simulink model "two_dof_system"  (R2019a)
settings: Solver=VariableStepAuto  StartTime=0.0  StopTime=time_span(end)  RelTol=1e-3
values from neighbouring files (symbols this model uses):
  c_f = damping    [cost_function.m]    (also in fourier_transform_two_dof_free.m = 100; two_dof_system_free_oscillations.m = 100)
  c_r = damping    [cost_function.m]    (also in fourier_transform_two_dof_free.m = 100; two_dof_system_free_oscillations.m = 100)
  j = 1000    [cost_function.m]    (also in fourier_transform_two_dof_free.m; two_dof_system_free_oscillations.m)
  k_f = 60000    [cost_function.m]    (also in fourier_transform_two_dof_free.m; two_dof_system_free_oscillations.m)
  k_r = 60000    [cost_function.m]    (also in fourier_transform_two_dof_free.m; two_dof_system_free_oscillations.m)
  l_f = 2.5    [cost_function.m]    (also in fourier_transform_two_dof_free.m; two_dof_system_free_oscillations.m = 4.5)
  l_r = 2.5    [cost_function.m]    (also in fourier_transform_two_dof_free.m; two_dof_system_free_oscillations.m)
  m = 1000    [cost_function.m]    (also in fourier_transform_two_dof_free.m; two_dof_system_free_oscillations.m)
  p_0 = 1.0    (= 1)    [cost_function.m]    (also in fourier_transform_two_dof_free.m; two_dof_system_free_oscillations.m)
  p_dot_0 = 0    [cost_function.m]    (also in fourier_transform_two_dof_free.m; two_dof_system_free_oscillations.m)
  x_0 = 0.1    [cost_function.m]    (also in fourier_transform_two_dof_free.m; two_dof_system_free_oscillations.m)
  x_dot_0 = 0    [cost_function.m]    (also in fourier_transform_two_dof_free.m; two_dof_system_free_oscillations.m)
settings Model: Creator=HP  LastModifiedBy=HP

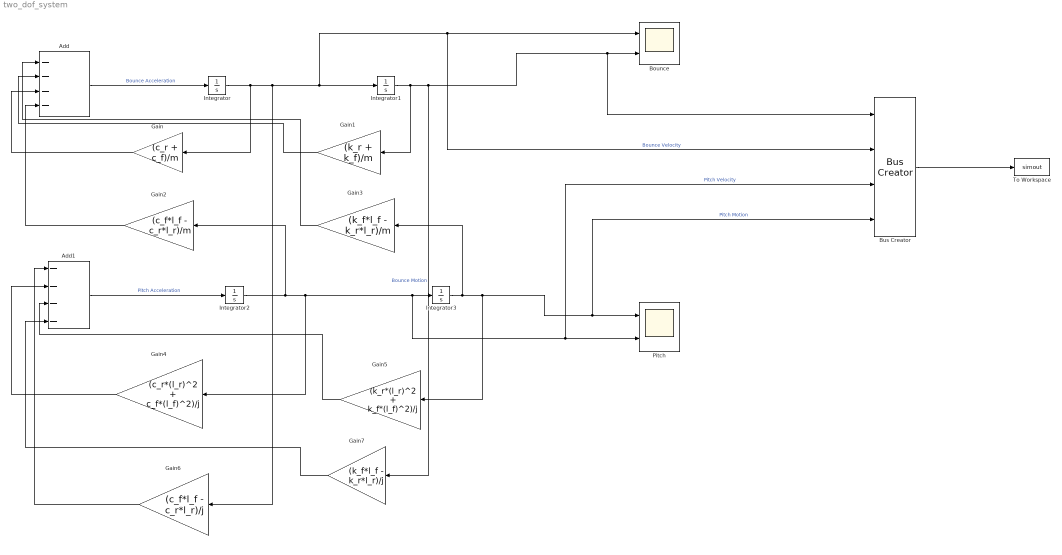
== system two_dof_system ==
  Add : Sum  Inputs=----
  Add1 : Sum  Inputs=----
  Bounce : Scope  NumInputPorts=2
  Bus Creator : BusCreator  Inputs=4
  Gain : Gain  Gain=(c_r + c_f)/m
  Gain1 : Gain  Gain=(k_r + k_f)/m
  Gain2 : Gain  Gain=(c_f*l_f - c_r*l_r)/m
  Gain3 : Gain  Gain=(k_f*l_f - k_r*l_r)/m
  Gain4 : Gain  Gain=(c_r*(l_r)^2 + c_f*(l_f)^2)/j
  Gain5 : Gain  Gain=(k_r*(l_r)^2 + k_f*(l_f)^2)/j
  Gain6 : Gain  Gain=(c_f*l_f - c_r*l_r)/j
  Gain7 : Gain  Gain=(k_f*l_f - k_r*l_r)/j
  Integrator : Integrator  InitialCondition=x_dot_0
  Integrator1 : Integrator  InitialCondition=x_0
  Integrator2 : Integrator  InitialCondition=p_dot_0
  Integrator3 : Integrator  InitialCondition=p_0
  Pitch : Scope  NumInputPorts=2
  To Workspace : ToWorkspace  VariableName=simout  SaveFormat=Timeseries  SampleTime=-1
  wires:
  Add/1 -> Integrator/1  "Bounce Acceleration"
  Integrator/1 -> Gain/1, Gain6/1, Bus Creator/2, Bounce/1, Integrator1/1  "Bounce Velocity"
  Integrator1/1 -> Gain1/1, Gain7/1, Bus Creator/1, Bounce/2  "Bounce Motion"
  Add1/1 -> Integrator2/1  "Pitch Acceleration"
  Integrator2/1 -> Gain2/1, Gain4/1, Bus Creator/3, Pitch/2, Integrator3/1  "Pitch Velocity"
  Integrator3/1 -> Gain3/1, Gain5/1, Bus Creator/4, Pitch/1  "Pitch Motion"
  Gain2/1 -> Add/4
  Gain/1 -> Add/3
  Gain1/1 -> Add/2
  Gain3/1 -> Add/1
  Gain6/1 -> Add1/1
  Gain4/1 -> Add1/2
  Gain5/1 -> Add1/3
  Gain7/1 -> Add1/4
  Bus Creator/1 -> To Workspace/1
